simulink model "Final_EV_2"  (R2024b)
settings: Solver=VariableStepAuto  StartTime=0  StopTime=inf  RelTol=1e-3
undefined symbols (not defined in the file): f
libraries: fl_lib x5, sdl_lib x5, nesl_utility x4, ee_lib x3, slrealtimeutilitieslib x1, simulink x1, autolibshared x1, instrumentlib x1
settings Model: Creator=User  LastModifiedBy=HP ELITEBOOK

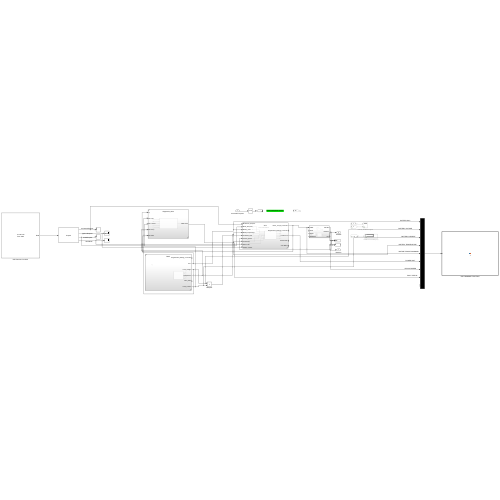
[thumbnail: Simulink's stored preview of the top-level diagram]
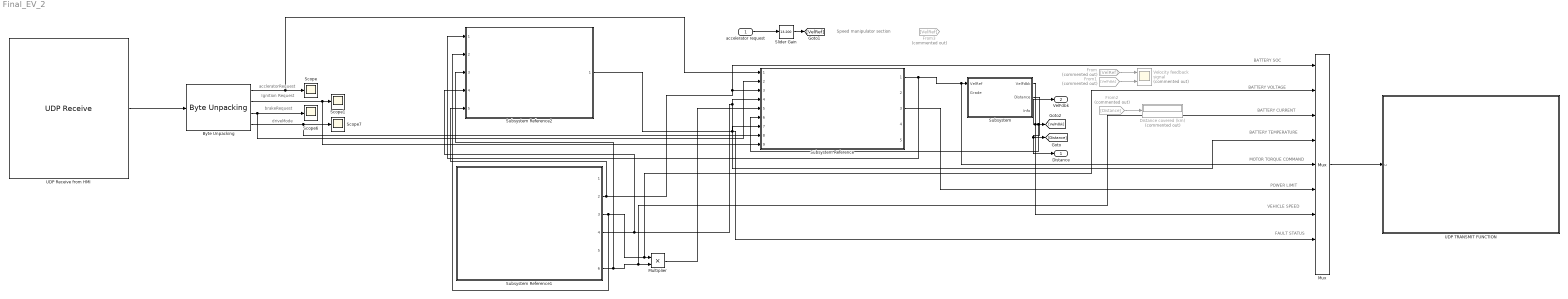
== system Final_EV_2 ==
  note: driveMode
  note: brakeRequest
  note: Ignition Request
  note: accleratorRequest
  note: FAULT STATUS
  note: VEHICLE SPEED
  note: POWER LIMIT
  note: MOTOR TORQUE COMMAND
  note: BATTERY TEMPERATURE
  note: BATTERY CURRENT
  note: BATTERY VOLTAGE
  note: BATTERY SOC
  note: Speed manipulator section
  accelerator request : Inport
  Byte Unpacking : slrealtimeutilitieslib/Byte Unpacking  MaskUnpackedDataTypes={'double', 'boolean', 'double', 'int32' }  MaskUnpackedDataSizes={[1], [1], [1], [1]}  MaskAlignment=1
  Distance covered (km) : Display  Commented=on
  From : From  Commented=on  GotoTag=VelRef
  From1 : From  Commented=on  GotoTag=VelFdbk
  From2 : From  Commented=on  GotoTag=Distance
  From3 : From  Commented=on  GotoTag=VelRef
  Multiplier : Product
  Mux : Mux  Inputs=9
  Scope{,1,6..7} (4 alike) : Scope
  Slider Gain : simulink/Math Operations/Slider Gain  gain=13.200  low=0  high=20
  Subsystem : Subsystem
  Subsystem Reference : Subsystem  ReferencedSubsystem=VCU
  Subsystem Reference1 : Subsystem  ReferencedSubsystem=BMS
  Subsystem Reference2 : Subsystem  ReferencedSubsystem=diagnostics_2024
  "UDP Receive from HMI " : instrumentlib/UDP Receive  LocalAddress=10.2.60.152  LocalPort=5000  EnablePortSharing=on  Host=localhost  Port=9090  GetLatestData=off  DataSize=[ 21, 1 ]  DataType=uint8  ASCIIFormatting=%f,  Terminator=LF  CustomTerminator=10  ByteOrder=little-endian  EnableBlockingMode=on  Timeout=10  SampleTime=0.01  SimulateUsing=Interpreted execution
  UDP TRANSMIT FUNCTION : MATLAB Function  TreatAsAtomicUnit=on
  Velocity feedback signal : Scope  Commented=on  NumInputPorts=2
  Distance : Outport
  VelFdbk : Outport  Port=2
  wires:
  accelerator request/1 -> Slider Gain/1
  From/1 -> Velocity feedback signal/1
  From1/1 -> Velocity feedback signal/2
  From2/1 -> Distance covered (km)/1
  Subsystem/2(Distance) -> Distance/1, [Distance]
  Slider Gain/1 -> [VelRef]
  Subsystem/1(VelFdbk) -> Subsystem Reference/6, [VelFdbk], VelFdbk/1, Mux/7
  Subsystem Reference1/2 -> Subsystem Reference2/5, Mux/1, Subsystem Reference/3
  Subsystem Reference1/4 -> Subsystem Reference2/4, Mux/4, Subsystem Reference/4
  Subsystem Reference/1 -> Subsystem Reference2/1, Mux/5, Subsystem/1(VelRef)
  Subsystem Reference1/3 -> Subsystem Reference2/2, Mux/2, Multiplier/1
  Subsystem Reference1/6 -> Subsystem Reference2/3, Multiplier/2, Mux/3
  Multiplier/1 -> Subsystem Reference/5
  Subsystem Reference2/1 -> Mux/8, Subsystem Reference/7
  Mux/1 -> UDP TRANSMIT FUNCTION/1(u)
  Subsystem Reference/3 -> Mux/6
  Byte Unpacking/2 -> Subsystem Reference/9, Scope1/1
  Byte Unpacking/3 -> Subsystem Reference/2, Scope6/1
  Byte Unpacking/1 -> Subsystem Reference/1, Scope/1
  "UDP Receive from HMI "/1 -> Byte Unpacking/1
  Byte Unpacking/4 -> Subsystem Reference/8, Scope7/1

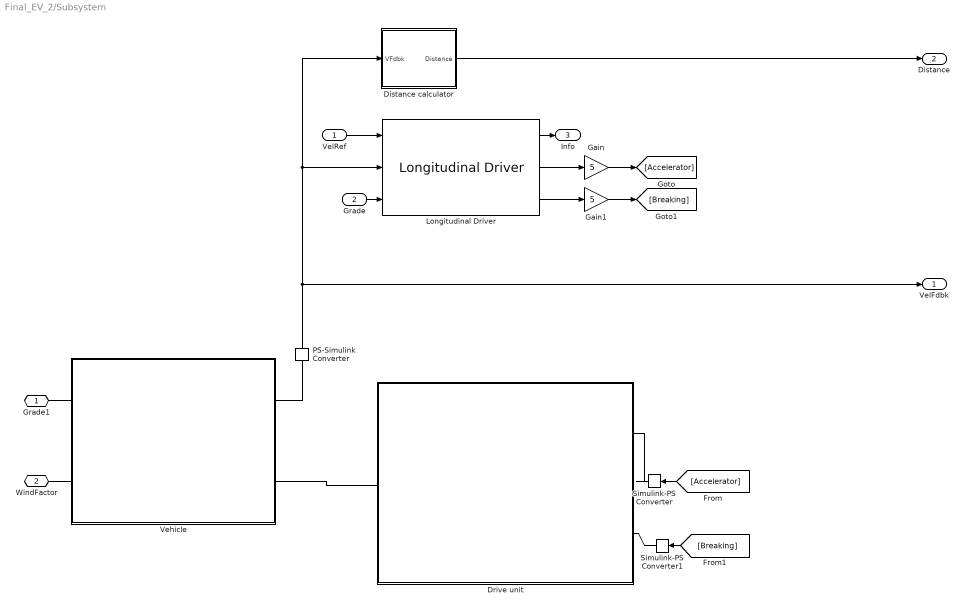
== system Final_EV_2/Subsystem ==
  VelRef : Inport
  Grade : Inport  Port=2
  Distance calculator : Subsystem
  Drive unit : Subsystem
  Gain : Gain  Gain=5
  Gain1 : Gain  Gain=5
  Longitudinal Driver : autolibshared/Longitudinal Driver  extAccelOvr=off  extDecelOvr=off  extAccelHld=off  extDecelHld=off  extAccelZero=off  extDecelZero=off  cntrlType=PI  shftType=None  velUnits=m/s  gearOut=off  Kp=150  Ki=100  Kff=.05  Kg=.01  VehVelVec=[0 100]  KffVec=[.1 .1]  KpVec=[10 10]  KiVec=[5 5]  KgVec=[0 0]  m=1600  Kpt=3000  tau=.1  L=2  aR=200  bR=2.5  cR=.5  g=9.81  vnom=100  Kaw=.1  tauerr=.03  tauPt=2  GearInit=0  tShift=.1  pdlVec=[0.1 0.4 0.5 0.9]  upShftTbl=[-1 12.9375 26.4375 39.9375 51.18749999999999 62.4375 72.84375 83.25;-1 16.3125 29.8125 43.3125 54.5624 65.8125 76.78125 87.75;-1 19.6875 33.1875 46.68749999999999 57.9375 69.1875 80.71875 92.25;-1 33 52.5 77.25 100.5 138.75 161.875 185]  dwnShftTbl=[1 9.5625 23.0625 36.5625 47.8125 59.0625 68.90625 78.75;1 12.9375 26.4375 39.9375 51.18749999999999 62.4375 72.84375 83.25;1 16.3125 29.8125 43.3125 54.562499 65.8125 76.78125 87.75;1 19.6875 33.1875 46.68749999999999 57.9375 69.1875 80.71875 92.25]  tClutch=.5  tRev=.5  tPark=120  aMode=1  UpGearVec="[0  1  2  3  4  5  6  7]"  DownGearVec="[1  2  3  4  5  6  7  8]"
  PS-Simulink Converter : nesl_utility/PS-Simulink Converter  PhysicalDomain=network_engine_domain  SubClassName=ps_output  LeftPortType=input  RightPortType=output  PseudoPeriodic=off  Frequencies=[]  VectorFormat=inherit  Unit=inherit  AffineConversion=off
  Simulink-PS Converter : nesl_utility/Simulink-PS Converter  PhysicalDomain=network_engine_domain  SubClassName=ps_input  LeftPortType=input  RightPortType=output  PseudoPeriodic=off  Frequencies=[]  NoiseDistribution=none  NoiseParameters=[]  Unit=1  AffineConversion=off  FilteringAndDerivatives=provide  SimscapeFilterOrder=1  InputFilterTimeConstant=0.001  UdotUserProvided=0
  Simulink-PS Converter1 : nesl_utility/Simulink-PS Converter  PhysicalDomain=network_engine_domain  SubClassName=ps_input  LeftPortType=input  RightPortType=output  PseudoPeriodic=off  Frequencies=[]  NoiseDistribution=none  NoiseParameters=[]  Unit=1  AffineConversion=off  FilteringAndDerivatives=provide  SimscapeFilterOrder=1  InputFilterTimeConstant=0.001  UdotUserProvided=0
  Vehicle : Subsystem
  Grade1 : PMIOPort  Side=Left
  WindFactor : PMIOPort  Port=2  Side=Left
  VelFdbk : Outport
  Distance : Outport  Port=2
  Info : Outport  Port=3
  wires:
  Gain/1 -> [Accelerator]
  [Breaking] -> Simulink-PS Converter1/1
  PS-Simulink Converter/1 -> VelFdbk/1, Distance calculator/1(VFdbk), Longitudinal Driver/2
  Gain1/1 -> [Breaking]
  Longitudinal Driver/3 -> Gain1/1
  Longitudinal Driver/2 -> Gain/1
  [Accelerator] -> Simulink-PS Converter/1
  Grade/1 -> Longitudinal Driver/3
  VelRef/1 -> Longitudinal Driver/1
  Distance calculator/1(Distance) -> Distance/1
  Longitudinal Driver/1 -> Info/1
  connections:
  Simulink-PS Converter1/RConn1 -- Drive unit/RConn2
  Vehicle/RConn2 -- Drive unit/LConn1
  Vehicle/RConn1 -- PS-Simulink Converter/LConn1
  Simulink-PS Converter/RConn1 -- Drive unit/RConn1
  Vehicle/LConn1 -- Grade1/RConn1
  Vehicle/LConn2 -- WindFactor/RConn1

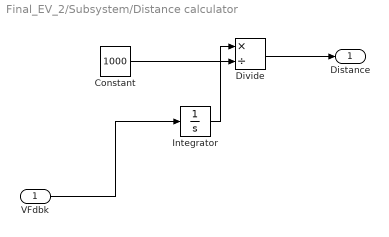
== system Final_EV_2/Subsystem/Distance calculator ==
  VFdbk : Inport
  Constant : Constant  Value=1000
  Divide : Product  Inputs=*/
  Integrator : Integrator
  Distance : Outport
  wires:
  Constant/1 -> Divide/2
  Integrator/1 -> Divide/1
  Divide/1 -> Distance/1
  VFdbk/1 -> Integrator/1

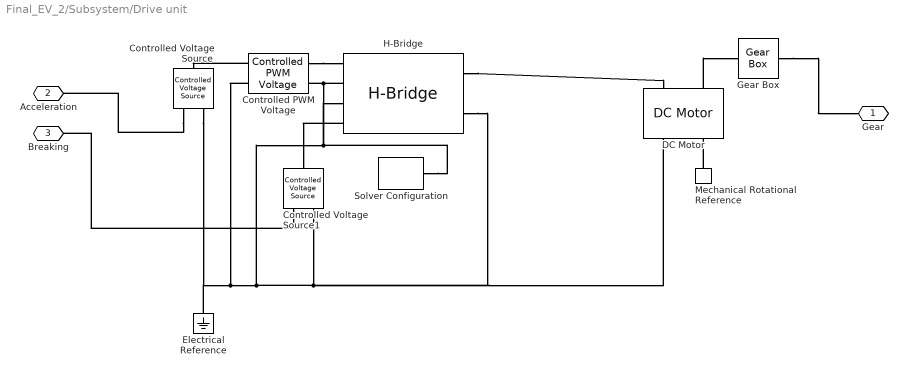
== system Final_EV_2/Subsystem/Drive unit ==
  Controlled PWM Voltage : ee_lib/Integrated Circuits/Controlled PWM Voltage  F=1000 Hz  TD=0 s  pulse_width_offset=0 s  pulse_min=0 s  pwm_or_av=ee.enum.pwm_or_av.averaged  event_type=ee.enum.ic.event.asynchronous  sample_time=1e-6 s  Vmin=0 V  Vmax=5 V  Vm=5 V  u_min=0  u_max=1
  Controlled Voltage Source : fl_lib/Electrical/Electrical Sources/Controlled Voltage Source
  Controlled Voltage Source1 : fl_lib/Electrical/Electrical Sources/Controlled Voltage Source
  DC Motor : ee_lib/Electromechanical/Brushed Motors/DC Motor  field_option=ee.enum.field_option.pm  Rf=100 Ohm  Lf=1 H  Laf=0.15 H  If0=0 A  parameterization=ee.enum.dcparam_option.load_speed  Ra=0.1 Ohm  La=100e-6 H  emf_or_torque=ee.enum.emf_or_torque.kv  Kv=0.08 V/rpm  Ki=6.876e-4 N*m/A  T_stall=300 N*m  w_max=5000 rpm  w_rated=3500 rpm  P_rated=110 kW  V_rated=370 V  lam_param=ee.enum.lam_param.damping  i_noload=0 A  V_i_noload=1.5 V  J=0.01 cm^2*g  lam=0 N*m*s/rad  speed0=0 rpm  t_fault_armature=1 s  t_fault_field=1 s  fault_action=simscape.enum.assert.action.none  alpha=3.93e-3 1/K  Tmeas=25 degC  thermal_mass=100 J/K  initial_temperature=25 degC
  Electrical Reference : fl_lib/Electrical/Electrical Elements/Electrical Reference
  Gear Box : fl_lib/Mechanical/Mechanisms/Gear Box  ratio=5  t_in_specify=off  t_in_priority=None  t_in=0 N*m  t_in_nominal_specify=off  t_in_nominal_value=1  t_in_nominal_unit=N*m  t_out_specify=off  t_out_priority=None  t_out=0 N*m  t_out_nominal_specify=off  t_out_nominal_value=1  t_out_nominal_unit=N*m
  H-Bridge : ee_lib/Semiconductors & Converters/Converters/H-Bridge  supply_ports=ee.enum.supply_ports.hidesupply  pwm_or_av=ee.enum.pwm_or_av.averaged  regenerative_braking_mode=ee.enum.converters.regenerative_braking_mode.always_enabled  discontinuous=ee.enum.current_profile.continuous  freewheeling_mode=ee.enum.converters.freewheeling_mode.one_switch_one_diode  Rload=10 Ohm  Lload=1e-5 H  F=10 kHz  Venable=2 V  Vmax=3.3 V  Vreverse=2 V  Vbrake=3.3 V  Vm=360 V  Ron=0.1 Ohm  Don=0.05 Ohm  Goff=1e-6 S  Tmeas=298.15 K  Ron2=0.1 Ohm  Don2=0.05 Ohm  Tmeas2=398.15 K  thermal_mass=100 J/K  initial_temperature=298.15 K
  Mechanical Rotational Reference : fl_lib/Mechanical/Rotational Elements/Mechanical Rotational Reference
  Solver Configuration : nesl_utility/Solver Configuration  PhysicalDomain=network_engine_domain  SubClassName=solver  LeftPortType=input  RightPortType=generic  Tones=[]  Harmonics=[]  SimulateNoise=off  Profile=off  UseLocalSampling=off  EnableSwitchedLinearOptims=on  FrequencyDomain=off  UseCCode=off  RelTol=0.001  AbsTol=0.001  MinStep=1e-09  ToWorkspace=off  RevertToSquareIcSolve=off  NumHomotopyIterations=100  PhasorMode=off  PhasorModeNumHarmonics=1  ConsistencySolver=NEWTON_XTOL_AFTER_FTOL  IndexReductionMethod=DerivativeReplacement  DoDC=off  ResidualTolerance=1e-09  ConsistencyTolSource=GLOBAL  ConsistencyAbsTol=0.001  ConsistencyRelTol=0.001  ConsistencyTolFactor=0.001  UseLocalSolver=off  LocalSolverChoice=NE_BACKWARD_EULER_ADVANCER  ResolveIndetEquations=on  FunctionEvalNumThread=1  LocalSolverSampleTime=0.001  DoFixedCost=off  MaxNonlinIter=3  MaxModeIter=2  ComputeImpulses=off  ImpulseIterations=2  LinearAlgebra=auto  LinearAlgebraNumThread=0  EquationFormulation=NE_TIME_EF  DelaysMemoryBudget=1024  AutomaticFiltering=on  FilteringTimeConstant=0.001  PartitionStorageMethod=AS_NEEDED  PartitionMemoryBudget=1024  PartitionMethod=ROBUST  MultibodyUseLocalSolver=off  MultibodyLocalSolverChoice=ODE1  MultibodyLocalSolverSampleTime=0.001
  Gear : PMIOPort  Side=Left
  Acceleration : PMIOPort  Port=2  Side=Right
  Breaking : PMIOPort  Port=3  Side=Right
  connections:
  H-Bridge/LConn2 -- Controlled Voltage Source1/RConn2 -- H-Bridge/RConn2 -- DC Motor/RConn1 -- Controlled Voltage Source/RConn2 -- Electrical Reference/LConn1 -- Controlled PWM Voltage/LConn2 -- Solver Configuration/RConn1 -- H-Bridge/LConn3 -- Controlled PWM Voltage/RConn2
  H-Bridge/LConn4 -- Controlled Voltage Source1/LConn1
  Controlled Voltage Source1/RConn1 -- Breaking/RConn1
  DC Motor/LConn2 -- Gear Box/LConn1
  Controlled PWM Voltage/RConn1 -- H-Bridge/LConn1
  Controlled PWM Voltage/LConn1 -- Controlled Voltage Source/LConn1
  Controlled Voltage Source/RConn1 -- Acceleration/RConn1
  Mechanical Rotational Reference/LConn1 -- DC Motor/RConn2
  Gear Box/RConn1 -- Gear/RConn1
  H-Bridge/RConn1 -- DC Motor/LConn1

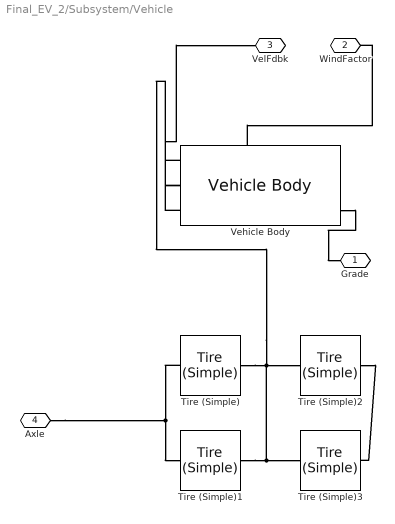
== system Final_EV_2/Subsystem/Vehicle ==
  Tire (Simple){,1..3} (4 alike) : sdl_lib/Tires & Vehicles/Tire (Simple)  r_tire=0.3 m  model_compliance=sdl.enum.compliance.off  stiffness=1e6 N/m  damping=1000 N*s/m  model_inertia=sdl.enum.model_inertia.off  tire_inertia=1 kg*m^2  initial_velocity=0 rad/s
      settings: InternalSimscapePortConfiguration="{\"Bottom\":[],\"Left\":[{\"id\":\"A\",\"label\":\"A\",\"type\":\"foundation.mechanical.rotational.rotational\"}],\"Right\":[{\"id\":\"H\",\"label\":\"H\",\"type\":\"foundation.mechanical.translational.translational\"}],\"Top\":[]}"
  Vehicle Body : sdl_lib/Tires & Vehicles/Vehicle Body  mass=1200 kg  n_w=2  x_f=1.4 m  x_r=1.6 m  y_c=0.5 m  mass_var=simscape.enum.onoff.off  g=9.81 m/s^2  liftoff_warning=simscape.enum.onoff.off  area=3 m^2  Cd_var=false  Cd=0.4  rho=1.18 kg/m^3  model_pitch=simscape.enum.onoff.off  inertia=4000 kg*m^2  suspension_model=sdl.enum.linearTLU.linear  k_f=1e4 N/m  b_f=1e4 N*s/m  k_r=1e4 N/m  b_r=1e4 N*s/m  k_f_TLU=[-2000, -1000, 0, 1000, 2000] N  x_f_TLU=[-.4, -.2, 0, .2, .4] m  b_f_TLU=[-200, -100, 0, 100, 200] N  v_f_TLU=[-4, -2, 0, 2, 4] m/s  k_r_TLU=[-2000, -1000, 0, 1000, 2000] N  x_r_TLU=[-.4, -.2, 0, .2, .4] m  b_r_TLU=[-200, -100, 0, 100, 200] N  v_r_TLU=[-4, -2, 0, 2, 4] m/s  interp_method=simscape.enum.interpolation.linear  extrap_method=simscape.enum.extrapolation.linear  model_hardstop=simscape.enum.onoff.off  upper_bound_f=.25 m  lower_bound_f=-.25 m  stop_k_f=1e6 N/m  stop_b_f=150 N*s/m  upper_bound_r=.25 m  lower_bound_r=-.25 m  stop_k_r=1e6 N/m  stop_b_r=150 N*s/m  initial_pitch=0 rad  initial_pitch_rate=0 rad/s  v_specify=off  v_priority=High  v=0 m/s  v_nominal_specify=off  v_nominal_value=1  v_nominal_unit=m/s
      settings: InternalSimscapePortConfiguration="{\"Bottom\":[{\"id\":\"NR\",\"label\":\"NR\",\"type\":\"output\"},{\"id\":\"NF\",\"label\":\"NF\",\"type\":\"output\"},{\"id\":\"beta\",\"label\":\"beta\",\"type\":\"input\"}],\"Left\":[{\"id\":\"H\",\"label\":\"H\",\"type\":\"foundation.mechanical.translational.translational\"}],\"Right\":[],\"Top\":[{\"id\":\"V\",\"label\":\"V\",\"type\":\"output\"},{\"id\":\"wind\",\"label\":\"W\",\"type\":\"input\"}]}"
  Grade : PMIOPort  Side=Left
  WindFactor : PMIOPort  Port=2  Side=Left
  VelFdbk : PMIOPort  Port=3  Side=Right
  Axle : PMIOPort  Port=4  Side=Right
  connections:
  Vehicle Body/LConn3 -- WindFactor/RConn1
  Vehicle Body/LConn2 -- VelFdbk/RConn1
  Vehicle Body/RConn3 -- Grade/RConn1
  Tire (Simple)1/RConn1 -- Vehicle Body/LConn1 -- Tire (Simple)2/RConn1 -- Tire (Simple)/RConn1 -- Tire (Simple)3/RConn1
  Tire (Simple)2/LConn1 -- Tire (Simple)3/LConn1
  Tire (Simple)/LConn1 -- Axle/RConn1 -- Tire (Simple)1/LConn1

== matlab function Final_EV_2/UDP TRANSMIT FUNCTION ==
  data: u input
function fcn(u)
% fcn - Sends Simulink telemetry data over UDP at every simulation step.
% u: Input vector from Simulink containing your telemetry variables.

% Declare the UDP object as persistent so it stays open between simulation steps
persistent uSender

% 1. Initialization (Runs ONLY on the very first time step)
if isempty(uSender)
    % Configure your target destination IP and Port here
    targetIP = "127.0.0.1"; % Change to your target's IP address
    targetPort = 9000;      % Change to your target's UDP port
    
    % Initialize the UDP port object
    uSender = udpport("LocalHost", "DestinationAddress", targetIP, "DestinationPort", targetPort);
end

% 2. Telemetry Processing & Packaging (Optional)
% If you need to convert your data to bytes, uint8, or apply an offset, do it here.
% For this example, we send the raw double vector directly.
packetData = double(u); 

% 3. Transmit Data
% "double" tells MATLAB to send the data as 8-byte floating-point numbers
write(uSender, packetData, "double");

end
